simulink model "Trial"  (R2021b)
settings: Solver=VariableStepAuto  StartTime=0.0  StopTime=1  RelTol=1e-3
values from neighbouring files (symbols this model uses):
  Ts = 2e-6    (= 2e-06)    [Para_Trial.m]
  Tsc = 5e-5    (= 5e-05)    [Para_Trial.m]
undefined symbols (not defined in the file or in its folder): CtrlMode, p
libraries: ee_lib x3, fl_lib x3, nesl_utility x2, eeTransforms x2, spsDCVoltageSourceLib x1, eePmsmFieldOrientedControl x1, eePmsmCurrentController x1, eePmsmCurrentReferenceGen x1, eeVelocityController x1, eePwmGeneratorTwoLevel x1, spsPermanentMagnetSynchronousMachineLib x1, spspowerguiLib x1
settings Model: Creator=Patron  LastModifiedBy=PurohitP
settings SolverCC: ZeroCrossAlgorithm=Adaptive
settings DebuggingCC: IgnoredZcDiagnostic=none

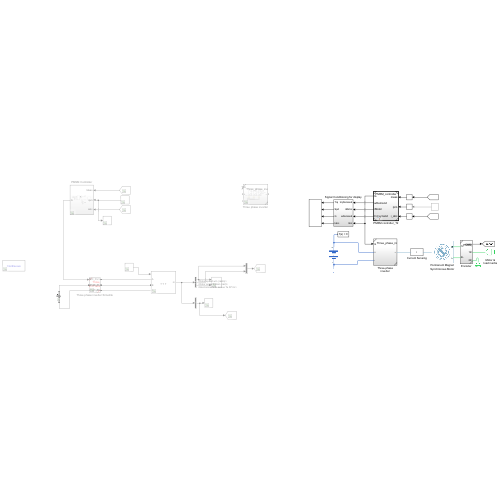
[thumbnail: Simulink's stored preview of the top-level diagram]
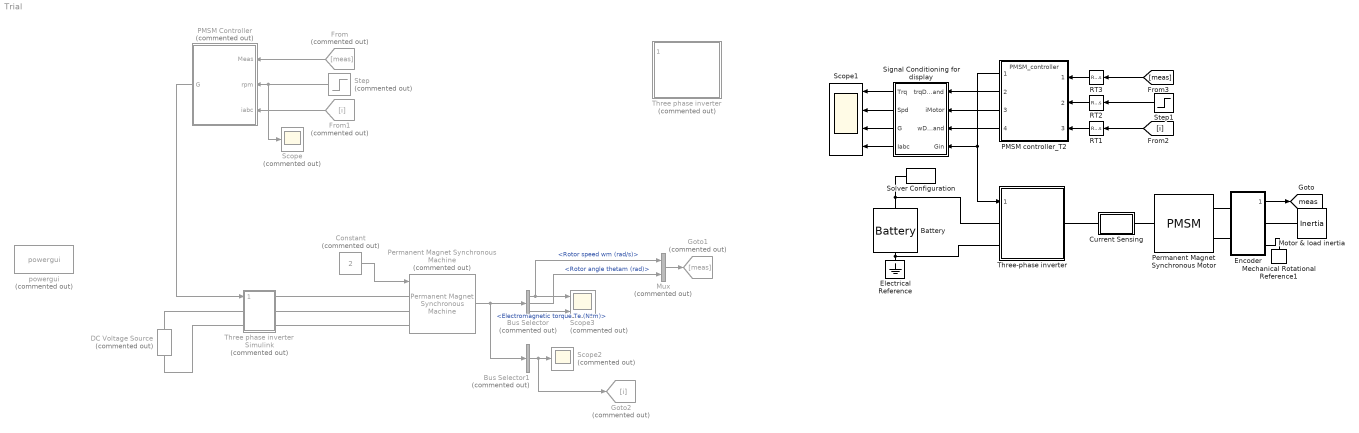
== system Trial ==
  Battery : ee_lib/Sources/Battery  Vnom=48 V  prm_dir=1  R1_dis=2 Ohm  R1_ch=2 Ohm  R1=0.001 Ohm  prm_AH=1  AH=14000 hr*A  V1=470 V  AH1=5000 hr*A  prm_R2=1  R2=inf Ohm  prm_dyn=1  Rp1=0.005 Ohm  tau1=30 s  Rp2=0.005 Ohm  tau2=30 s  Rp3=0.005 Ohm  tau3=30 s  Rp4=0.005 Ohm  tau4=30 s  Rp5=0.005 Ohm  tau5=30 s  prm_fade=1  N_fade=100  AH_fade=45 hr*A  R1_fade=2.02 Ohm  R1_ch_fade=2.02 Ohm  V1_fade=10.35 V  prm_age=1  prm_age_OCV=1  OCV_age=0.9  SOC_age=60  delta_time_age_vec=[0] d  temperature_age_vec=[273] K  OCV_scaling_age=2.2134e6  OCV_offset_age=1.632e6  temp_exp_age=0.515833569 V  t_exp_age=0.75  i_specify=off  i_priority=None  i=0 A  i_nominal_specify=off  i_nominal_unit=A  i_nominal_value=1  v_specify=off  v_priority=None  v=0 V  v_nominal_specify=off  v_nominal_unit=V  v_nominal_value=1  charge_specify=on  charge_priority=High  charge=7000 hr*A  charge_nominal_specify=off  charge_nominal_unit=hr*A  charge_nominal_value=1  num_cycles_specify=off  num_cycles_priority=High  num_cycles=0  num_cycles_nominal_specify=off  num_cycles_nominal_unit=1  num_cycles_nominal_value=1  Tmeas=298.15 K  Tmeas_age=298.15 K  Vnom_T2=12 V  R1_T2=2.2 Ohm  R1_T2_dis=2.2 Ohm  R1_T2_ch=2.2 Ohm  V1_T2=11.4 V  R2_T2=2200 Ohm  Rp1_T2=0.005 Ohm  tau1_T2=30 s  Rp2_T2=0.005 Ohm  tau2_T2=30 s  Rp3_T2=0.005 Ohm  tau3_T2=30 s  Rp4_T2=0.005 Ohm  tau4_T2=30 s  Rp5_T2=0.005 Ohm  tau5_T2=30 s  Tmeas2=273.15 K  thermal_mass=30000 J/K  temperature_specify=off  temperature_priority=High  temperature=298.15 K  temperature_nominal_specify=off  temperature_nominal_unit=K  temperature_nominal_value=1
  Bus Selector : BusSelector  Commented=on  OutputSignals=Rotor speed wm (rad/s),Rotor angle thetam (rad),Electromagnetic torque Te (N*m)
  Bus Selector1 : BusSelector  Commented=on  OutputSignals=Stator current is_a (A),Stator current is_b (A),Stator current is_c (A)  OutputAsBus=on
  Constant : Constant  Commented=on  Value=2
  Current Sensing : Subsystem
      mask Display: disp('i')
  DC Voltage Source : spsDCVoltageSourceLib/DC Voltage Source  Commented=on  Amplitude=300  Measurements=None
  Electrical Reference : fl_lib/Electrical/Electrical Elements/Electrical Reference
  Encoder : Subsystem  ReferencedSubsystem=PMSM_Encoder
  From : From  Commented=on  GotoTag=meas
  From1 : From  Commented=on  GotoTag=i
  Goto1 : Goto  Commented=on  GotoTag=meas
  Goto2 : Goto  Commented=on  GotoTag=i
  Mechanical Rotational Reference1 : fl_lib/Mechanical/Rotational Elements/Mechanical Rotational Reference
  Motor & load inertia : fl_lib/Mechanical/Rotational Elements/Inertia  inertia=J kg*m^2  num_ports=foundation.enum.numPorts2.one  w_specify=on  w_priority=High  w=0 rpm  w_nominal_specify=off  w_nominal_unit=rad/s  w_nominal_value=1  t_specify=off  t_priority=High  t=0 N*m  t_nominal_specify=off  t_nominal_unit=N*m  t_nominal_value=1
  Mux : Mux  Commented=on  Inputs=2
  PMSM Controller : Subsystem  Commented=on
  PMSM controller_T2 : ModelReference  ModelNameDialog=PMSM_controller  SimulationMode=Normal  ModelReferenceVersion=1.73
  Permanent Magnet Synchronous Machine : spsPermanentMagnetSynchronousMachineLib/Permanent Magnet Synchronous Machine  Commented=on  NbPhases=3  FluxDistribution=Sinusoidal  RotorType=Round  MechanicalLoad=Torque Tm  PresetModel="06:  10 Nm 300 Vdc 2300 RPM - 14.2 Nm"  ShowDetailedParameters=on  MeasurementBus=off  Resistance=0.4578  Inductance=8.5e-3  dqInductances=[8.5e-3,8.5e-3]  La=0.00334  MachineConstant=Flux linkage established by magnets (V.s)  Flux=0.171  VoltageCst=124.0639  TorqueCst=1.026  Flat=120  Mechanical=[0.001469 0.0003035 4 0]  PolePairs=4  InitialConditions=[0,0, 0,0]  InitialConditions5ph=[0 0 0 0 0 0]  RefAngle=90 degrees behind phase A axis (modified Park)  IterativeDiscreteModel=Trapezoidal non iterative  TsBlock=-1  TsPowergui=0
  Permanent Magnet Synchronous Motor : ee_lib/Electromechanical/Permanent Magnet/PMSM  port_option=ee.enum.threePhasePort.composite  winding_type=ee.enum.statorconnection.wye  machine_param=ee.enum.pmsm.parameterization.constant  nPolePairs=N  pmflux_param=ee.enum.pmflux.fluxlinkage  pm_flux_linkage=PM Wb  torque_constant=0.18 N*m/A  back_emf_constant=0.18 V/(rad/s)  stator_param=ee.enum.statorparam.LdLqL0  Ld=Ld H  Lq=Lq H  idVec=[-200, 0, 200] A  iqVec=[-200, 0, 200] A  LdMatrix=0.0002 * ones(3, 3) H  LqMatrix=0.0002 * ones(3, 3) H  PmMatrix=0.1 * ones(3, 3) Wb  ktMatrix=0.18 * ones(3, 3) N*m/A  keMatrix=0.18 * ones(3, 3) V/(rad/s)  L0=L0 H  Ls=0.0002 H  Lm=0.00002 H  Ms=0.00002 H  Rs=Rs Ohm  zero_sequence=ee.enum.park.zerosequence.exclude  axes_param=ee.enum.rotorangle.qaxis  loss_param=ee.enum.ironloss.none  losses_oc=[0, 0, 0] W  losses_sc=[0, 0, 0] W  f_losses=60 Hz  Isc_losses=95 A  J=0 kg*m^2  lam=0 N*m/(rad/s)  i_d_specify=off  i_d_priority=None  i_d=0 A  i_d_nominal_specify=off  i_d_nominal_unit=A  i_d_nominal_value=1  i_q_specify=off  i_q_priority=None  i_q=0 A  i_q_nominal_specify=off  i_q_nominal_unit=A  i_q_nominal_value=1  torque_specify=off  torque_priority=None  torque=0 N*m  torque_nominal_specify=off  torque_nominal_unit=N*m  torque_nominal_value=1  angular_velocity_specify=on  angular_velocity_priority=None  angular_velocity=0 rpm  angular_velocity_nominal_specify=off  angular_velocity_nominal_unit=rpm  angular_velocity_nominal_value=1  angular_position_specify=on  angular_position_priority=High  angular_position=0 rad  angular_position_nominal_specify=off  angular_position_nominal_unit=deg  angular_position_nominal_value=1  alpha=3.93e-3 1/K  alpha_flux=-0.001 1/K  Tmeas=298.15 K  stator_thermal_mass=100 J/K  rotor_thermal_mass=200 J/K  Rm_percent_rotor=90  Rd_percent_rotor=30  temperatureA_specify=off  temperatureA_priority=High  temperatureA=25 degC  temperatureA_nominal_specify=off  temperatureA_nominal_unit=degC  temperatureA_nominal_value=1  temperatureB_specify=off  temperatureB_priority=High  temperatureB=25 degC  temperatureB_nominal_specify=off  temperatureB_nominal_unit=degC  temperatureB_nominal_value=1  temperatureC_specify=off  temperatureC_priority=High  temperatureC=25 degC  temperatureC_nominal_specify=off  temperatureC_nominal_unit=degC  temperatureC_nominal_value=1  temperatureR_specify=off  temperatureR_priority=High  temperatureR=25 degC  temperatureR_nominal_specify=off  temperatureR_nominal_unit=degC  temperatureR_nominal_value=1
      settings: InternalSimscapePortConfiguration="{\"Bottom\":[],\"Left\":[{\"id\":\"N\",\"label\":\"~\",\"type\":\"foundation.electrical.three_phase\"}],\"Right\":[{\"id\":\"R\",\"label\":\"R\",\"type\":\"foundation.mechanical.rotational.rotational\"},{\"id\":\"C\",\"label\":\"C\",\"type\":\"foundation.mechanical.rotational.rotational\"}],\"Top\":[]}"
  RT1 : RateTransition  OutPortSampleTime=Tsc
  RT2 : RateTransition  OutPortSampleTime=Tsc
  RT3 : RateTransition  OutPortSampleTime=Tsc
  Scope : Scope  Commented=on
  Scope1 : Scope  NumInputPorts=4
  Scope2 : Scope  Commented=on
  Scope3 : Scope  Commented=on  NumInputPorts=2
  Signal Conditioning for display : Subsystem
  Solver Configuration : nesl_utility/Solver Configuration  PhysicalDomain=network_engine_domain  SubClassName=solver  LeftPortType=input  RightPortType=generic  Tones=[]  Harmonics=[]  SimulateNoise=off  Profile=off  UseLocalSampling=off  EnableSwitchedLinearOptims=on  FrequencyDomain=off  UseCCode=off  RelTol=0.001  AbsTol=1e-06  MinStep=1e-09  ToWorkspace=off  RevertToSquareIcSolve=off  NumHomotopyIterations=100  PhasorMode=off  PhasorModeNumHarmonics=1  DoDC=off  ResidualTolerance=1e-9  UseLocalSolver=off  LocalSolverChoice=NE_BACKWARD_EULER_ADVANCER  LocalSolverSampleTime=Ts  DoFixedCost=off  MaxNonlinIter=4  MaxModeIter=2  ComputeImpulses=off  ImpulseIterations=2  LinearAlgebra=auto  EquationFormulation=NE_TIME_EF  DelaysMemoryBudget=1024  AutomaticFiltering=on  FilteringTimeConstant=0.001  PartitionStorageMethod=AS_NEEDED  PartitionMemoryBudget=1024  PartitionMethod=FAST
      settings: SourceProductBaseCode=PW,SS
  Step : Step  Commented=on  Time=0.1  After=8
  Step1 : Step  Time=0.1  After=200  SampleTime=0
  Three phase inverter : Subsystem  Commented=on  ReferencedSubsystem=Three_phase_inverter
  Three phase inverter Simulink : Subsystem  Commented=on  ReferencedSubsystem=Three_phase_inverter_Simulink
  Three-phase inverter : Subsystem  ReferencedSubsystem=Three_phase_inverter
  powergui : spspowerguiLib/powergui  Priority=1  Commented=on  SimulationMode=Continuous  SampleTime=5e-6  frequency=60  Iterations=50  frequencyindice=0  Pbase=100e6  ErrMax=1e-4  UnitsV=kV  UnitsW=MW  buscounter=0  FunctionMessages=off  echomessages=off  EnableUseOfTLC=off  CurrentSourceSwitches=off  DisableSnubberDevices=off  DisableRonSwitches=off  DisableVfSwitches=off  DisplayEquations=off  AutomaticDiscreteSolvers=off  SolverType=Tustin/Backward Euler (TBE)  Interpol=off  ExternalGateDelay=off  methode=off  Ts=100  x0status=blocks  SPID=on  SwTol=0  HookPort=off  NonlinearTolerance=1e-4  nMaxIteration=100  ContinueOnMaxIteration=off  RestoreLinks=warning  ResistiveCurrentMeasurement=off  Frange=[0:2:500]  Ylog=off  Xlog=on  ShowGrid=off  save=off  variable=ZData  structure=0  ZoomFFT=off  StartTime=0.0  cycles=1  DisplayStyle=1  fundamental=60  FreqAxis=off  MaxFrequency=1000  frequencyindicesteady=1  RmsSteady=1  display=off
  tag scope: meas=global
  wires:
  From/1 -> PMSM Controller/1(Meas)
  Step/1 -> Scope/1, PMSM Controller/2(rpm)
  From1/1 -> PMSM Controller/3(iabc)
  Constant/1 -> Permanent Magnet Synchronous Machine/1
  Permanent Magnet Synchronous Machine/1 -> Bus Selector1/1, Bus Selector/1
  Bus Selector1/1 -> Goto2/1, Scope2/1
  Bus Selector/1 -> Mux/1, Scope3/1  "<Rotor speed wm (rad/s)>"
  Bus Selector/3 -> Scope3/2  "<Electromagnetic torque Te (N*m)>"
  PMSM Controller/1(G) -> Three phase inverter Simulink/1
  Bus Selector/2 -> Mux/2  "<Rotor angle thetam (rad)>"
  Mux/1 -> Goto1/1
  Signal Conditioning for display/1(Trq) -> Scope1/1
  RT1/1 -> PMSM controller_T2/3
  RT3/1 -> PMSM controller_T2/1
  Signal Conditioning for display/4(Iabc) -> Scope1/4
  PMSM controller_T2/1 -> Three-phase inverter/1, Signal Conditioning for display/4(Gin)
  [i] -> RT1/1
  Signal Conditioning for display/3(G) -> Scope1/3
  RT2/1 -> PMSM controller_T2/2
  Signal Conditioning for display/2(Spd) -> Scope1/2
  Encoder/1 -> [meas]
  Step1/1 -> RT2/1
  [meas] -> RT3/1
  PMSM controller_T2/2 -> Signal Conditioning for display/1(trqDemand)
  PMSM controller_T2/3 -> Signal Conditioning for display/2(iMotor)
  PMSM controller_T2/4 -> Signal Conditioning for display/3(wDemand)
  connections:
  Permanent Magnet Synchronous Machine/LConn1 -- Three phase inverter Simulink/RConn1
  Permanent Magnet Synchronous Machine/LConn2 -- Three phase inverter Simulink/RConn2
  Permanent Magnet Synchronous Machine/LConn3 -- Three phase inverter Simulink/RConn3
  DC Voltage Source/RConn1 -- Three phase inverter Simulink/LConn1
  DC Voltage Source/LConn1 -- Three phase inverter Simulink/LConn2
  Battery/LConn1 -- Three-phase inverter/LConn1 -- Solver Configuration/RConn1
  Battery/RConn1 -- Three-phase inverter/LConn2 -- Electrical Reference/LConn1
  Mechanical Rotational Reference1/LConn1 -- Encoder/RConn2
  Current Sensing/LConn1 -- Three-phase inverter/RConn1
  Encoder/RConn1 -- Motor & load inertia/LConn1
  Permanent Magnet Synchronous Motor/RConn1 -- Encoder/LConn1
  Permanent Magnet Synchronous Motor/RConn2 -- Encoder/LConn2
  Permanent Magnet Synchronous Motor/LConn1 -- Current Sensing/RConn1

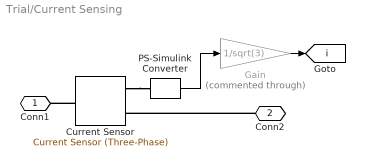
== system Trial/Current Sensing ==
  Current Sensor : ee_lib/Sensors & Transducers/Current Sensor (Three-Phase)
  Gain : Gain  Commented=through  Gain=1/sqrt(3)
  PS-Simulink Converter : nesl_utility/PS-Simulink Converter  PhysicalDomain=network_engine_domain  SubClassName=ps_output  LeftPortType=input  RightPortType=output  PseudoPeriodic=off  Frequencies=[]  Unit=A  AffineConversion=off
      settings: SourceProductBaseCode=PW,SS
  Conn1 : PMIOPort  Side=Left
  Conn2 : PMIOPort  Port=2  Side=Right
  tag scope: i=global
  wires:
  PS-Simulink Converter/1 -> Gain/1
  Gain/1 -> [i]
  connections:
  Current Sensor/RConn1 -- PS-Simulink Converter/LConn1
  Conn2/RConn1 -- Current Sensor/RConn2
  Current Sensor/LConn1 -- Conn1/RConn1

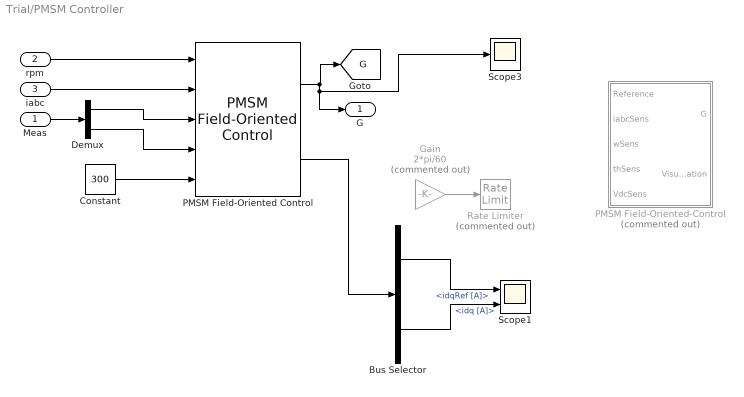
== system Trial/PMSM Controller ==
  Meas : Inport
  rpm : Inport  Port=2
  iabc : Inport  Port=3
  Bus Selector : BusSelector  OutputSignals=idqRef [A],idq [A]
  Constant : Constant  Value=300
  Demux : Demux  Outputs=2
  Gain : Gain  Commented=on  Gain=2*pi/60
  PMSM Field-Oriented Control : eePmsmFieldOrientedControl/PMSM Field-Oriented Control  winding_type=Wye-wound  CtrlMode=Torque control  Vnom=300  Pmax=23000  Tmax=14.2  p=4  Vdc_on=6  Ts=5e-6  Tsc=1e-4  CtrlType=PI control  Kp_w=1  Ki_w=100  Kv_w=1  Kaw_w=1  RefType=Zero d-axis control  rpmVec=[0, 3000]  TqVec=[-100, 0, 100]  VdcVec=[300, 350]  PWMMode=SVM: space vector modulation  ModFactor=1  idMatrix=zeros(2,3,2)  iqMatrix=zeros(2,3,2)  psim=0.171  Ld=0.00024  Lq=0.00029  Rs=0.01  AxisAlignment=Q-axis  Kp_id=0.01  Ki_id=100  Kaw_id=0  Kp_iq=0.01  Ki_iq=100  Kaw_iq=0  AxisPrio=Q-axis  ActZC=off  ActFF=on  ParamTypeFF=Constant parameters  LdFF=0.00334  LqFF=0.00334  psimFF=0.171  idVect=[-200, 0, 200]  iqVect=[-200, 0, 200]  LdMatrix=0.0002 * ones(3, 3)  LqMatrix=0.0002 * ones(3, 3)  psimMatrix=0.04 * ones(3, 3)  CPWMMode=SVM: space vector modulation  fsw=10000
      settings: SourceProductBaseCode=PS
  PMSM Field-Oriented-Control : Subsystem  Commented=on
  Rate Limiter : RateLimiter  Commented=on  SampleTimeMode=inherited
  Scope1 : Scope  NumInputPorts=2
  Scope3 : Scope
  G : Outport
  tag scope: G=global
  wires:
  Meas/1 -> Demux/1
  Gain/1 -> Rate Limiter/1
  iabc/1 -> PMSM Field-Oriented Control/2
  Demux/1 -> PMSM Field-Oriented Control/3
  Demux/2 -> PMSM Field-Oriented Control/4
  Constant/1 -> PMSM Field-Oriented Control/5
  PMSM Field-Oriented Control/1 -> G/1, Scope3/1, [G]
  rpm/1 -> PMSM Field-Oriented Control/1
  Bus Selector/1 -> Scope1/1  "<idqRef [A]>"
  Bus Selector/2 -> Scope1/2  "<idq [A]>"
  PMSM Field-Oriented Control/2 -> Bus Selector/1

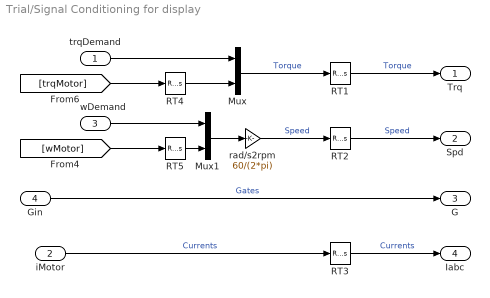
== system Trial/Signal Conditioning for display ==
  trqDemand : Inport
  iMotor : Inport  Port=2
  wDemand : Inport  Port=3
  Gin : Inport  Port=4
  Mux : Mux  Inputs=2
  Mux1 : Mux  Inputs=2
  RT1 : RateTransition  OutPortSampleTime=Ts
  RT2 : RateTransition  OutPortSampleTime=Ts
  RT3 : RateTransition  OutPortSampleTime=Ts
  RT4 : RateTransition  OutPortSampleTime=Tsc
  RT5 : RateTransition  OutPortSampleTime=Tsc
  rad/s2rpm : Gain  Gain=60/(2*pi)
  Trq : Outport  VectorParamsAs1DForOutWhenUnconnected=off
  Spd : Outport  Port=2  VectorParamsAs1DForOutWhenUnconnected=off
  G : Outport  Port=3  VectorParamsAs1DForOutWhenUnconnected=off
  Iabc : Outport  Port=4  VectorParamsAs1DForOutWhenUnconnected=off
  wires:
  trqDemand/1 -> Mux/1
  Gin/1 -> G/1  "Gates"
  Mux1/1 -> rad/s2rpm/1
  Mux/1 -> RT1/1  "Torque"
  iMotor/1 -> RT3/1  "Currents"
  wDemand/1 -> Mux1/1
  rad/s2rpm/1 -> RT2/1  "Speed"
  [trqMotor] -> RT4/1
  [wMotor] -> RT5/1
  RT1/1 -> Trq/1  "Torque"
  RT2/1 -> Spd/1  "Speed"
  RT3/1 -> Iabc/1  "Currents"
  RT4/1 -> Mux/2
  RT5/1 -> Mux1/2

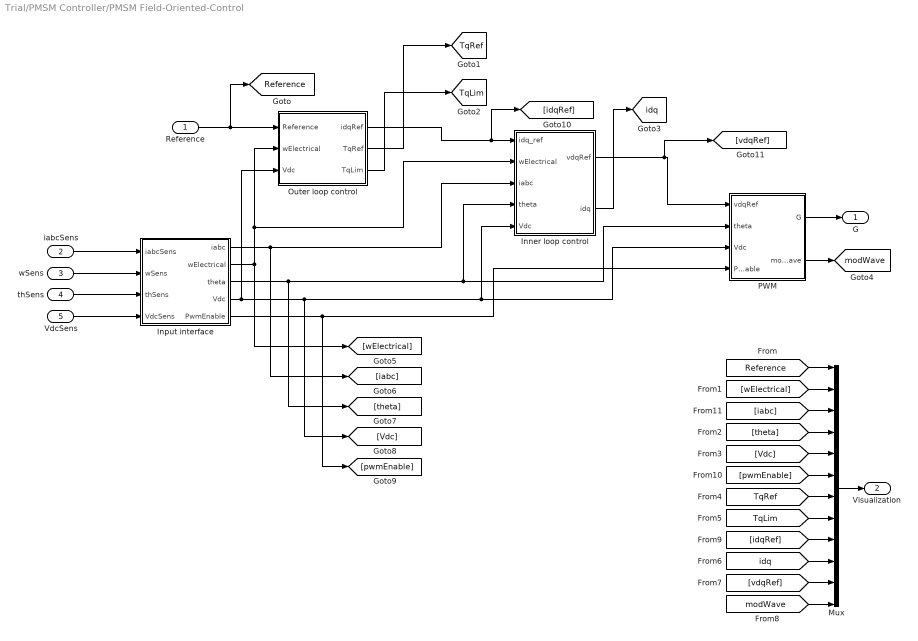
== system Trial/PMSM Controller/PMSM Field-Oriented-Control ==
  Reference : Inport
  iabcSens : Inport  Port=2
  wSens : Inport  Port=3
  thSens : Inport  Port=4
  VdcSens : Inport  Port=5
  Inner loop control : Subsystem
  Input interface : Subsystem
  Mux : Mux  Inputs=12
  Outer loop control : Subsystem
  PWM : Subsystem
  G : Outport
  Visualization : Outport  Port=2
  tag scope: Reference=global, TqLim=global, TqRef=global, idq=global, modWave=global
  wires:
  Reference/1 -> [Reference], Outer loop control/1(Reference)
  iabcSens/1 -> Input interface/1(iabcSens)
  wSens/1 -> Input interface/2(wSens)
  VdcSens/1 -> Input interface/4(VdcSens)
  thSens/1 -> Input interface/3(thSens)
  Input interface/2(wElectrical) -> Inner loop control/2(wElectrical), Outer loop control/2(wElectrical), [wElectrical]
  Input interface/1(iabc) -> [iabc], Inner loop control/3(iabc)
  Input interface/5(PwmEnable) -> [pwmEnable], PWM/4(PWMEnable)
  Input interface/3(theta) -> [theta], Inner loop control/4(theta), PWM/2(theta)
  Inner loop control/1(vdqRef) -> [vdqRef], PWM/1(vdqRef)
  Outer loop control/1(idqRef) -> [idqRef], Inner loop control/1(idq_ref)
  Input interface/4(Vdc) -> [Vdc], Inner loop control/5(Vdc), PWM/3(Vdc), Outer loop control/3(Vdc)
  Outer loop control/2(TqRef) -> [TqRef]
  Outer loop control/3(TqLim) -> [TqLim]
  Inner loop control/2(idq) -> [idq]
  PWM/1(G) -> G/1
  PWM/2(modWave) -> [modWave]
  Mux/1 -> Visualization/1
  [Reference] -> Mux/1
  [wElectrical] -> Mux/2
  [theta] -> Mux/4
  [Vdc] -> Mux/5
  [TqRef] -> Mux/7
  [TqLim] -> Mux/8
  [idq] -> Mux/10
  [vdqRef] -> Mux/11
  [modWave] -> Mux/12
  [idqRef] -> Mux/9
  [pwmEnable] -> Mux/6
  [iabc] -> Mux/3

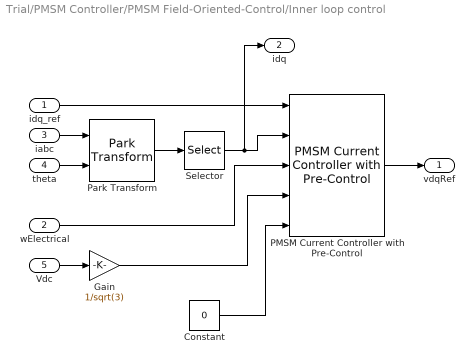
== system Trial/PMSM Controller/PMSM Field-Oriented-Control/Inner loop control ==
  idq_ref : Inport
  wElectrical : Inport  Port=2
  iabc : Inport  Port=3
  theta : Inport  Port=4
  Vdc : Inport  Port=5
  Constant : Constant  Value=0
  Gain : Gain  Gain=1/sqrt(3)
  PMSM Current Controller with Pre-Control : eePmsmCurrentController/PMSM Current Controller with Pre-Control  Kp_id=1  Ki_id=100  Kaw_id=1  Kp_iq=1  Ki_iq=100  Kaw_iq=1  Ts=-1  Tsd=0.001  AxisPrio=Q-axis  ActZC=off  ActFF=on  idVect=[-200, 0, 200]  iqVect=[-200, 0, 200]  LdMatrix=0.0002 * ones(3, 3)  LqMatrix=0.0002 * ones(3, 3)  psimMatrix=0.04 * ones(3, 3)
      settings: SourceProductBaseCode=PS
  Park Transform : eeTransforms/Park Transform  AxisAlignment=Q-axis  PowerInvariant=off
  Selector : Selector  InputPortWidth=3  IndexOptions=Index vector (dialog)  Indices=[1 2]  OutputSizes=1
  vdqRef : Outport
  idq : Outport  Port=2
  wires:
  idq_ref/1 -> PMSM Current Controller with Pre-Control/1
  iabc/1 -> Park Transform/1
  theta/1 -> Park Transform/2
  Park Transform/1 -> Selector/1
  Selector/1 -> idq/1, PMSM Current Controller with Pre-Control/2
  wElectrical/1 -> PMSM Current Controller with Pre-Control/3
  Vdc/1 -> Gain/1
  Gain/1 -> PMSM Current Controller with Pre-Control/4
  Constant/1 -> PMSM Current Controller with Pre-Control/5
  PMSM Current Controller with Pre-Control/1 -> vdqRef/1

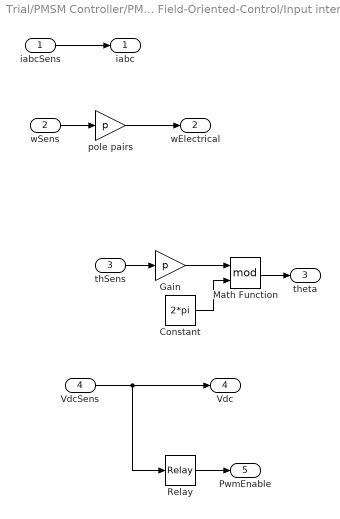
== system Trial/PMSM Controller/PMSM Field-Oriented-Control/Input interface ==
  iabcSens : Inport
  wSens : Inport  Port=2
  thSens : Inport  Port=3
  VdcSens : Inport  Port=4
  Constant : Constant  Value=2*pi
  Gain : Gain  Gain=p
  Math Function : Math  Operator=mod  SaturateOnIntegerOverflow=on
  Relay : Relay
  pole pairs : Gain  Gain=p
  iabc : Outport
  wElectrical : Outport  Port=2
  theta : Outport  Port=3
  Vdc : Outport  Port=4
  PwmEnable : Outport  Port=5
  wires:
  wSens/1 -> pole pairs/1
  pole pairs/1 -> wElectrical/1
  thSens/1 -> Gain/1
  Gain/1 -> Math Function/1
  Constant/1 -> Math Function/2
  Math Function/1 -> theta/1
  VdcSens/1 -> Relay/1, Vdc/1
  iabcSens/1 -> iabc/1
  Relay/1 -> PwmEnable/1

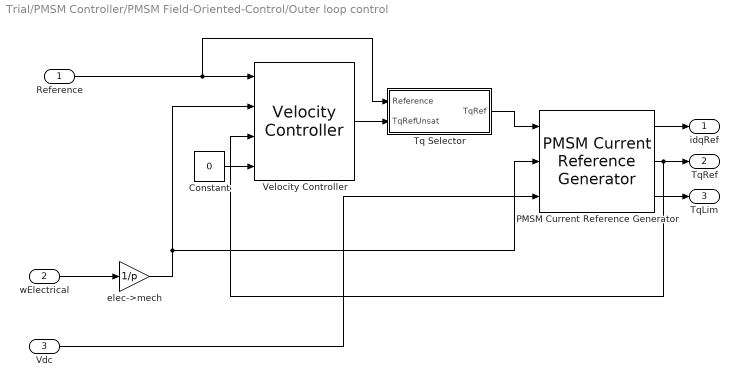
== system Trial/PMSM Controller/PMSM Field-Oriented-Control/Outer loop control ==
  Reference : Inport
  wElectrical : Inport  Port=2
  Vdc : Inport  Port=3
  Constant : Constant  Value=0
  PMSM Current Reference Generator : eePmsmCurrentReferenceGen/PMSM Current Reference Generator  Vnom=300  Pmax=30000  Tmax=250  Ts=Tsc  RefType=Zero d-axis control  rpmVec=[0, 3000]  TqVec=[-100, 0, 100]  VdcVec=[300, 350]  PWMMode=SVM: space vector modulation  ModFactor=1  idMatrix=zeros(2,3,2)  iqMatrix=zeros(2,3,2)  p=8  psim=0.04  Ld=0.00024  Lq=0.00029  Rs=0.01  RefExpEnable=0
      settings: SourceProductBaseCode=PS
  Tq Selector : Subsystem
  Velocity Controller : eeVelocityController/Velocity Controller  CtrlType=PI control  Kp_w=1  Ki_w=1  Kv_w=1  Kaw_w=1  Ts=-1  Tsd=0.001  ActZC=off
      settings: SourceProductBaseCode=PS
  elec->mech : Gain  Gain=1/p
  idqRef : Outport
  TqRef : Outport  Port=2
  TqLim : Outport  Port=3
  wires:
  wElectrical/1 -> elec->mech/1
  Reference/1 -> Tq Selector/1(Reference), Velocity Controller/1
  elec->mech/1 -> PMSM Current Reference Generator/2, Velocity Controller/2
  Constant/1 -> Velocity Controller/4
  Velocity Controller/1 -> Tq Selector/2(TqRefUnsat)
  Tq Selector/1(TqRef) -> PMSM Current Reference Generator/1
  Vdc/1 -> PMSM Current Reference Generator/3
  PMSM Current Reference Generator/1 -> idqRef/1
  PMSM Current Reference Generator/2 -> Velocity Controller/3, TqRef/1
  PMSM Current Reference Generator/3 -> TqLim/1

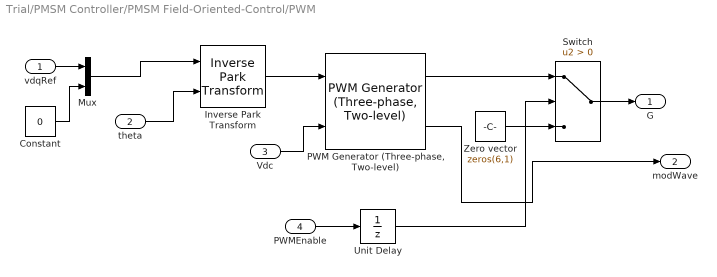
== system Trial/PMSM Controller/PMSM Field-Oriented-Control/PWM ==
  vdqRef : Inport
  theta : Inport  Port=2
  Vdc : Inport  Port=3
  PWMEnable : Inport  Port=4
  Constant : Constant  Value=0
  Inverse Park Transform : eeTransforms/Inverse Park Transform  AxisAlignment=Q-axis  PowerInvariant=off
  Mux : Mux  Inputs=2
  "PWM Generator (Three-phase, Two-level)" : eePwmGeneratorTwoLevel/PWM Generator (Three-phase, Two-level)  PWMMode=Continuous PWM (CPWM)  CPWMMode=SPWM: sinusoidal PWM  DPWMMode=60 DPWM: 60 degree discontinuous PWM  fsw=1e3  Ts=5e-5
      settings: SourceProductBaseCode=PS
  Switch : Switch  Criteria=u2 > Threshold
  Unit Delay : UnitDelay  SampleTime=Tsc  HasFrameUpgradeWarning=on
  Zero vector : Constant  Value=zeros(6,1)  SampleTime=Ts
  G : Outport
  modWave : Outport  Port=2
  wires:
  Inverse Park Transform/1 -> "PWM Generator (Three-phase, Two-level)"/1
  vdqRef/1 -> Mux/1
  Constant/1 -> Mux/2
  Mux/1 -> Inverse Park Transform/1
  theta/1 -> Inverse Park Transform/2
  Vdc/1 -> "PWM Generator (Three-phase, Two-level)"/2
  PWMEnable/1 -> Unit Delay/1
  Unit Delay/1 -> Switch/2
  "PWM Generator (Three-phase, Two-level)"/1 -> Switch/1
  Zero vector/1 -> Switch/3
  Switch/1 -> G/1
  "PWM Generator (Three-phase, Two-level)"/2 -> modWave/1

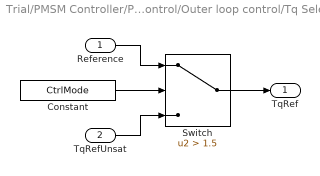
== system Trial/PMSM Controller/PMSM Field-Oriented-Control/Outer loop control/Tq Selector ==
  Reference : Inport
  TqRefUnsat : Inport  Port=2
  Constant : Constant  Value=CtrlMode  SampleTime=Tsc
  Switch : Switch  Criteria=u2 > Threshold  Threshold=1.5
  TqRef : Outport
  wires:
  Constant/1 -> Switch/2
  Reference/1 -> Switch/1
  Switch/1 -> TqRef/1
  TqRefUnsat/1 -> Switch/3
